simulink model "Pacemaker_A2_02_workingSerial"  (R2020a)
settings: Solver=FixedStepAuto  StartTime=0.0  StopTime=10.0  FixedStep=1e-3  RelTol=1e-3  EnableMultiTasking=on
undefined symbols (not defined in the file): D0, D1, D10, D11, D12, D13, D2, D3, D4, D5, D6, D7, D8, D9, PTA0, PTA1, PTA2, PTB23, PTB9, PTC16, PTC17, PTC2, PTC3, PTC4, PTD0, PTD1, PTD2, PTD3
libraries: frdmk64flib x22, etargetslib x2
settings Model: ExtModeTrigDuration=5  Creator=forre  LastModifiedBy=forre
settings OptimizationCC: EnhancedBackFolding=on  PassReuseOutputArgsAs=Individual arguments  ZeroExternalMemoryAtStartup=off  ZeroInternalMemoryAtStartup=off  MaxStackSize=64  OptimizeBlockOrder=speed  DifferentSizesBufferReuse=on  OptimizationCustomize=off  EfficientTunableParamExpr=on
settings DebuggingCC: ParameterTunabilityLossMsg=error
settings HardwareCC: ProdBitPerPointer=32  ProdBitPerSizeT=32  ProdBitPerPtrDiffT=32  ProdLargestAtomicInteger=Long  ProdLargestAtomicFloat=Double  ProdWordSize=32  ProdHWDeviceType=ARM Compatible->ARM Cortex
settings SFSimCC: MATLABDynamicMemAlloc=off
settings RTWCC: SystemTargetFile=ert.tlc  HardwareBoard=NXP FRDM-K64F  TemplateMakefile=ert_default_tmf  Toolchain=GNU Tools for ARM Embedded Processors
settings CodeAppCC: ForceParamTrailComments=on  IgnoreCustomStorageClasses=off  OperatorAnnotations=on  SimulinkDataObjDesc=on  SFDataObjDesc=on  InsertBlockDesc=on

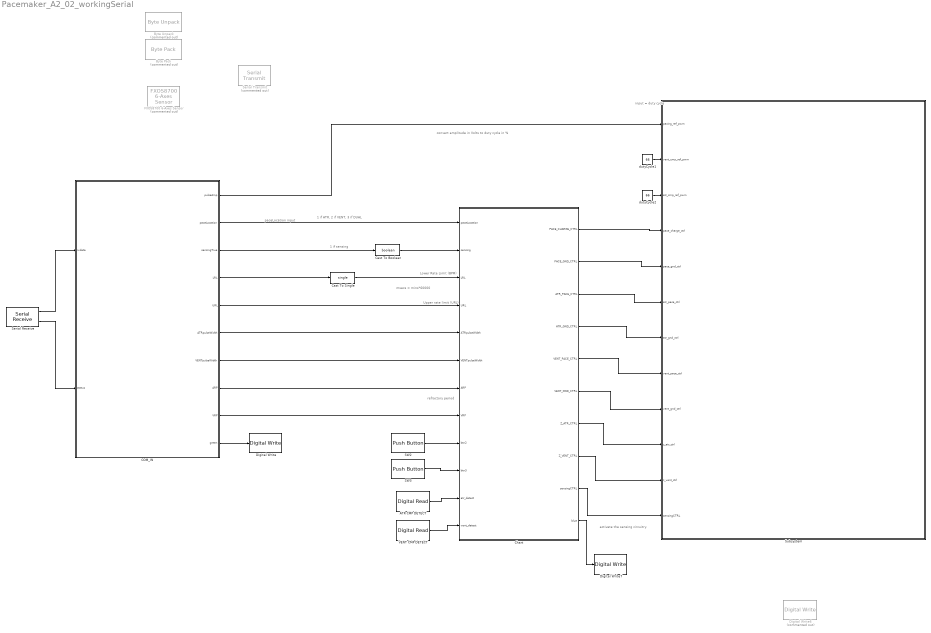
== system Pacemaker_A2_02_workingSerial ==
  note: convert amplitude in Volts to duty cycle in %
  note: msecs = mins*60000
  note: Upper rate limit (URL)
  note: refractory period
  note: Lower Rate Limit (BPM)
  note: paceLocation input
  note: activate the sensing circuitry.
  note: 1 if ATR, 2 if VENT, 3 if DUAL
  note: input = duty cycle
  note: 1 if sensing
  ATR CMP DETECT : frdmk64flib/Digital Read  Whichpin=PTC16 (D0)  SampleTime=-1
  Byte Pack : etargetslib/Byte Pack  Commented=on  datatypes={'single'}  byteAlign=1
  Byte Unpack : etargetslib/Byte Unpack  Commented=on  dimensions={[1]}  datatypes={'double'}  byteAlign=1
  COM_IN : Stateflow chart  TreatAsAtomicUnit=on
  Cast To Boolean : DataTypeConversion  OutDataTypeStr=boolean
  Cast To Single : DataTypeConversion  OutDataTypeStr=single
  Chart : Stateflow chart  TreatAsAtomicUnit=on
  Digital Write : frdmk64flib/Digital Write  Whichpin=GREEN_LED
  Digital Write6 : frdmk64flib/Digital Write  Commented=on  Whichpin=RED_LED
  Digital Write7 : frdmk64flib/Digital Write  Whichpin=BLUE_LED
  FXOS8700 6-Axes Sensor : frdmk64flib/FXOS8700 6-Axes Sensor  Commented=on  Activesensor=Accelerometer only  ODR=800Hz  HybridODR=400Hz  Accelfullrange=-4g to +4g  SampleTime=-1
  SW2 : frdmk64flib/Push Button  Whichswitch=SW2  SampleTime1=-1
  SW3 : frdmk64flib/Push Button  Whichswitch=SW3  SampleTime1=-1
  Serial Receive : frdmk64flib/Serial Receive  SCIModule=0  Baudrate=uint32(9600)  Parity=None  StopBits=1  HardwareFlowControl=None  ByteOrder=LittleEndian  DataType=uint8  DataLength=30  BlockingMode=off  OutputStatus=on  SampleTime=-1
  Serial Transmit : frdmk64flib/Serial Transmit  Commented=on  SCIModule=0  Baudrate=uint32(9600)  Parity=None  StopBits=1  HardwareFlowControl=None  ByteOrder=LittleEndian  BlockingMode=on  OutputStatus=off
  Subsystem : Subsystem
  VENT CMP DETECT : frdmk64flib/Digital Read  Whichpin=PTC17 (D1)  SampleTime=-1
  dutyCycle1 : Constant  Value=66
  dutyCycle2 : Constant  Value=66
  wires:
  SW2/1 -> Chart/9(btn2)
  Chart/4(ATR_GND_CTRL) -> Subsystem/7(atr_gnd_ctrl)
  Chart/3(ATR_PACE_CTRL) -> Subsystem/6(atr_pace_ctrl)
  Chart/1(PACE_CHARGE_CTRL) -> Subsystem/4(pace_charge_ctrl)
  Chart/2(PACE_GND_CTRL) -> Subsystem/5(pace_gnd_ctrl)
  Chart/5(VENT_PACE_CTRL) -> Subsystem/8(vent_pace_ctrl)
  Chart/6(VENT_GND_CTRL) -> Subsystem/9(vent_gnd_ctrl)
  Chart/7(Z_ATR_CTRL) -> Subsystem/10(z_atr_ctrl)
  Chart/8(Z_VENT_CTRL) -> Subsystem/11(" z_vent_ctrl")
  ATR CMP DETECT/1 -> Chart/11(atr_detect)
  VENT CMP DETECT/1 -> Chart/12(vent_detect)
  dutyCycle1/1 -> Subsystem/2(vent_cmp_ref_pwm)
  dutyCycle2/1 -> Subsystem/3(atr_cmp_ref_pwm)
  Chart/9(sensingCTRL) -> Subsystem/12(sensingCTRL)
  COM_IN/3(sensingTrue) -> Cast To Boolean/1
  ? -> Digital Write6/1
  Chart/10(blue) -> Digital Write7/1
  SW3/1 -> Chart/10(btn3)
  COM_IN/5(URL) -> Chart/4(URL)
  COM_IN/8(ARP) -> Chart/7(ARP)
  COM_IN/9(VRP) -> Chart/8(VRP)
  Serial Receive/1 -> COM_IN/1(rxdata)
  Serial Receive/2 -> COM_IN/2(status)
  COM_IN/2(paceLocation) -> Chart/1(paceLocation)
  COM_IN/6(ATRpulseWidth) -> Chart/5(ATRpulseWidth)
  COM_IN/7(VENTpulseWidth) -> Chart/6(VENTpulseWidth)
  Cast To Boolean/1 -> Chart/2(sensing)
  COM_IN/4(LRL) -> Cast To Single/1
  Cast To Single/1 -> Chart/3(LRL)
  COM_IN/10(green) -> Digital Write/1
  COM_IN/1(pulseAmp) -> Subsystem/1(pacing_ref_pwm)

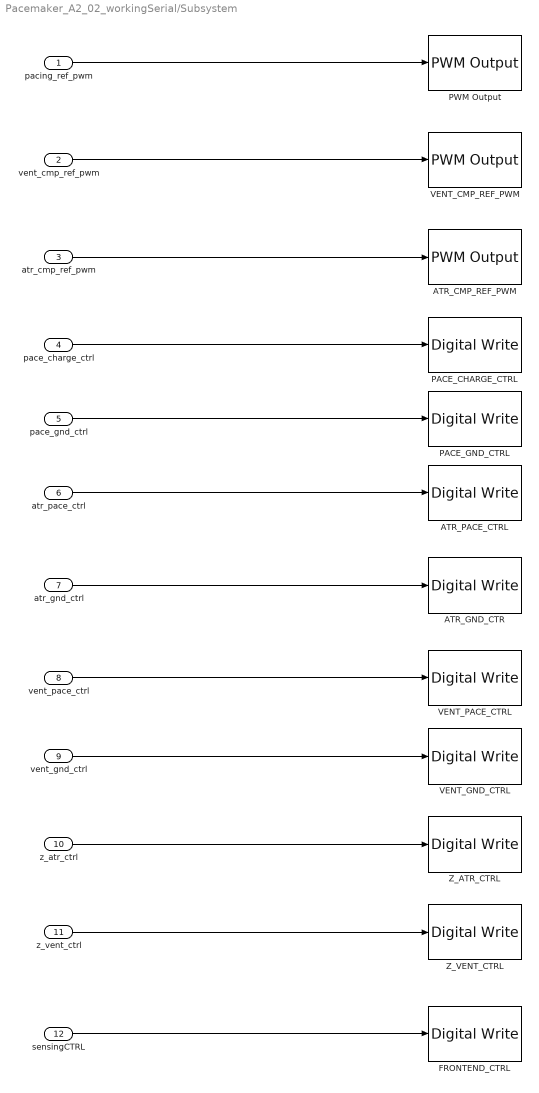
== system Pacemaker_A2_02_workingSerial/Subsystem ==
  pacing_ref_pwm : Inport
  vent_cmp_ref_pwm : Inport  Port=2
  atr_cmp_ref_pwm : Inport  Port=3
  pace_charge_ctrl : Inport  Port=4
  pace_gnd_ctrl : Inport  Port=5
  atr_pace_ctrl : Inport  Port=6
  atr_gnd_ctrl : Inport  Port=7
  vent_pace_ctrl : Inport  Port=8
  vent_gnd_ctrl : Inport  Port=9
  z_atr_ctrl : Inport  Port=10
  " z_vent_ctrl" : Inport  Port=11
  sensingCTRL : Inport  Port=12
  ATR_CMP_REF_PWM : frdmk64flib/PWM Output  Whichpin=PTC2 (D6)  InitialFrequency=2000  InitialDutyCycle=50
  ATR_GND_CTR : frdmk64flib/Digital Write  Whichpin=PTD2 (D11)
  ATR_PACE_CTRL : frdmk64flib/Digital Write  Whichpin=PTA0 (D8)
  FRONTEND_CTRL : frdmk64flib/Digital Write  Whichpin=PTD1 (D13)
  PACE_CHARGE_CTRL : frdmk64flib/Digital Write  Whichpin=PTB9 (D2)
  PACE_GND_CTRL : frdmk64flib/Digital Write  Whichpin=PTD0 (D10)
  PWM Output : frdmk64flib/PWM Output  Whichpin=PTA2 (D5)  InitialFrequency=2000  InitialDutyCycle=50
  VENT_CMP_REF_PWM : frdmk64flib/PWM Output  Whichpin=PTA1 (D3)  InitialFrequency=2000  InitialDutyCycle=50
  VENT_GND_CTRL : frdmk64flib/Digital Write  Whichpin=PTD3 (D12)
  VENT_PACE_CTRL : frdmk64flib/Digital Write  Whichpin=PTC4 (D9)
  Z_ATR_CTRL : frdmk64flib/Digital Write  Whichpin=PTB23 (D4)
  Z_VENT_CTRL : frdmk64flib/Digital Write  Whichpin=PTC3 (D7)
  wires:
  pace_gnd_ctrl/1 -> PACE_GND_CTRL/1
  atr_pace_ctrl/1 -> ATR_PACE_CTRL/1
  pace_charge_ctrl/1 -> PACE_CHARGE_CTRL/1
  atr_gnd_ctrl/1 -> ATR_GND_CTR/1
  vent_pace_ctrl/1 -> VENT_PACE_CTRL/1
  vent_gnd_ctrl/1 -> VENT_GND_CTRL/1
  z_atr_ctrl/1 -> Z_ATR_CTRL/1
  " z_vent_ctrl"/1 -> Z_VENT_CTRL/1
  sensingCTRL/1 -> FRONTEND_CTRL/1
  pacing_ref_pwm/1 -> PWM Output/1
  vent_cmp_ref_pwm/1 -> VENT_CMP_REF_PWM/1
  atr_cmp_ref_pwm/1 -> ATR_CMP_REF_PWM/1

== stateflow chart Pacemaker_A2_02_workingSerial/Chart ==
  note: beat sensed
  state SENSING_VENT_TRUE
    entry:
    sensingCTRL = true;
  state VENT_CHARGING_AND_DISCHARGE
    entry:
    % for this state paceLocation = 1
    %begin charge and discharge cycle for ventricle
    msecPerPace = 60000.0/LRL; %new value in msec
    sensingCTRL = sensing; %enables the sensing circuitry if sensing = 1. Controled by input "sensing"
    ATR_PACE_CTRL = false;
    VENT_PACE_CTRL = false;
    PACE_CHARGE_CTRL = true;
    PACE_GND_CTRL = true;
    Z_VENT_CTRL = false;
    Z_ATR_CTRL = false
    VENT_GND_CTRL = true;
    ATR_GND_CTRL = false;
  state VENT_PACING
    entry:
    % pace ventricle
    PACE_GND_CTRL = true;
    VENT_PACE_CTRL = true;
    VENT_GND_CTRL = false;
    Z_VENT_CTRL = false;
    Z_ATR_CTRL = false;
    ATR_GND_CTRL = false;
    ATR_PACE_CTRL = false;
    sensingCTRL = sensing; %enables the sensing circuitry if sensing = 1. Controled by input "sensing"
  note: VENT PACING
  note: switch to vent
  note: switch to atr
  state ATR_CHARGING_AND_DISCHARGE
    entry:
    % for this state paceLocation = 0
    %begin charge and discharge cycle for atrium
    msecPerPace = 60000.0/LRL; %new value for pace timing with msec units
    sensingCTRL = sensing; %enables the sensing circuitry if sensing = 1. Controled by input "sensing"
    ATR_PACE_CTRL = false;
    VENT_PACE_CTRL = false;
    PACE_CHARGE_CTRL = true;
    PACE_GND_CTRL = true;
    Z_VENT_CTRL = false;
    Z_ATR_CTRL = false;
    VENT_GND_CTRL = false;
    ATR_GND_CTRL = true;
    blue=false;
  state ATR_PACING
    entry:
    % pace atrium
    PACE_GND_CTRL = true;
    VENT_PACE_CTRL = false;
    VENT_GND_CTRL = false;
    Z_VENT_CTRL = false;
    Z_ATR_CTRL = false;
    ATR_GND_CTRL = false;
    ATR_PACE_CTRL = true;
    sensingCTRL = sensing; %enables the sensing circuitry if sensing = 1. Controled by input "sensing"
  note: ATR PACING
  state SENSING_ATR_TRUE
    entry:
    sensingCTRL = true;
  note: switch to atr
  note: beat sensed
  note: switch to dual
  state DUAL [commented out]
  VENT_PACING -> VENT_CHARGING_AND_DISCHARGE : after(VENTpulseWidth, msec)
  VENT_CHARGING_AND_DISCHARGE -> SENSING_VENT_TRUE [order 2] : after((VRP-VENTpulseWidth),msec)[sensing && (vent_detect || btn3)]
  SENSING_VENT_TRUE -> VENT_CHARGING_AND_DISCHARGE : after(VENTpulseWidth, msec)
  VENT_CHARGING_AND_DISCHARGE -> DUAL [commented out] : [paceLocation==3]
  DUAL -> VENT_CHARGING_AND_DISCHARGE [commented out]
  VENT_CHARGING_AND_DISCHARGE -> VENT_PACING [order 1] : after((msecPerPace-VENTpulseWidth), msec){PACE_CHARGE_CTRL = false;}
  ATR_CHARGING_AND_DISCHARGE -> VENT_CHARGING_AND_DISCHARGE [order 3] : [paceLocation==2]{blue=false;}
  VENT_CHARGING_AND_DISCHARGE -> ATR_CHARGING_AND_DISCHARGE [order 3] : [paceLocation==1]{blue=true;}
  (default) -> ATR_CHARGING_AND_DISCHARGE
  ATR_CHARGING_AND_DISCHARGE -> DUAL [commented out] : [paceLocation==3]
  ATR_CHARGING_AND_DISCHARGE -> ATR_PACING [order 1] : after((msecPerPace-ATRpulseWidth), msec){PACE_CHARGE_CTRL = false;}
  DUAL -> ATR_CHARGING_AND_DISCHARGE [commented out] : [paceLocation==1]
  ATR_PACING -> ATR_CHARGING_AND_DISCHARGE : after(ATRpulseWidth, msec)
  ATR_CHARGING_AND_DISCHARGE -> SENSING_ATR_TRUE [order 2] : after((ARP-ATRpulseWidth),msec)[sensing && (atr_detect || btn3)]
  SENSING_ATR_TRUE -> ATR_CHARGING_AND_DISCHARGE : after(ATRpulseWidth, msec)
  data: paceLocation input uint8; sensing input boolean; LRL input single; URL input uint8; ATRpulseWidth input single; VENTpulseWidth input single; ARP input single; VRP input single; PACE_CHARGE_CTRL output boolean; PACE_GND_CTRL output boolean; btn2 input boolean; btn3 input boolean; ATR_PACE_CTRL output boolean; ATR_GND_CTRL output boolean; msecPerBeat local single; VENT_PACE_CTRL output boolean; VENT_GND_CTRL output boolean; Z_ATR_CTRL output boolean; Z_VENT_CTRL output boolean; atr_detect input boolean; vent_detect input boolean; sensingCTRL output boolean; msecPerPace local single; blue output boolean
  data paceLocation settings: description=|
      | 0 = pace atrium
      | 1 = pace ventricle
  data atr_detect settings: description=|
      | 0 = pace atrium
      | 1 = pace ventricle
  data vent_detect settings: description=|
      | 0 = pace atrium
      | 1 = pace ventricle

== stateflow chart Pacemaker_A2_02_workingSerial/COM_IN ==
  state SET_PARAMETERS
    entry:
    paceLocation = rxdata(3); %1 if ATRIUM, 2 if VENT, 3 if BOTH
    sensingTrue = rxdata(4); %1 if sensing, 0 if not
    LRL = rxdata(5);
    URL =  rxdata(6);
    AtrAmp = typecast(rxdata(7:10), 'single');
    VentAmp = typecast(rxdata(11:14),'single');
    ATRpulseWidth = typecast(rxdata(15:18),'single');
    VENTpulseWidth = typecast(rxdata(19:22),'single');
    ARP = typecast(rxdata(23:26),'single');
    VRP = typecast(rxdata(27:30),'single');
  state INITIAL
    entry:
    paceLocation = 1;
    sensingTrue = 0; %1 if sensing, 0 if not
    LRL = 60;
    URL = 120;
    AtrAmp = 50;
    VentAmp = 50;
    ATRpulseWidth = 10;
    VENTpulseWidth = 10;
    ARP = 250;
    VRP = 250;
    green = false;
  state STANDBY
    %waiting
  state ECHO_PARAMETERS
    entry:
    %send_parameters();
  SET_PARAMETERS -> STANDBY [order 2] : [paceLocation==2]{pulseAmp = VentAmp;}
  SET_PARAMETERS -> STANDBY [order 1] : [paceLocation==1]{pulseAmp = AtrAmp;}
  (default) -> INITIAL
  (junction 14) -> SET_PARAMETERS [order 1] : [rxdata(2) == hex2dec('55')]
  (junction 18) -> STANDBY [order 2]
  INITIAL -> STANDBY
  STANDBY -> (junction 18) : [status==0]
  (junction 18) -> (junction 14) [order 1] : [rxdata(1) == hex2dec('16')]
  (junction 14) -> ECHO_PARAMETERS [order 2] : [rxdata(2) == hex2dec('22')]
  ECHO_PARAMETERS -> STANDBY
  data: pulseAmp output single; paceLocation output uint8; sensingTrue output uint8; LRL output uint8; URL output uint8; ATRpulseWidth output single; VENTpulseWidth output single; ARP output single; rxdata input uint8; VRP output single; status input uint8; green output boolean; AtrAmp local single; VentAmp local single
